simulink model "shuzi"  (Simulink 5.0)
settings: Solver=ode45  StartTime=0.0  StopTime=10.0  RelTol=1e-3
undefined symbols (not defined in the file): rcosine
libraries: dspsigops x6, simulink x3, commsink2 x2, commchan2 x1, commrandsrc2 x1, commutil2 x1, dspswit3 x1, dsparch4 x1, commcontsrc2 x1
settings Model: LastModifiedBy=lenovo

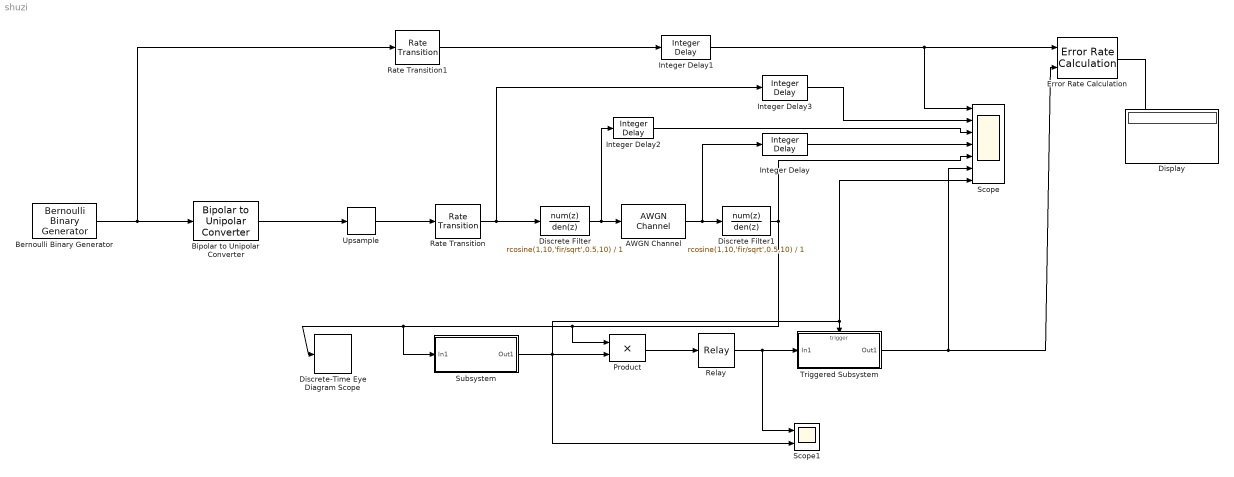
== system shuzi ==
  AWGN Channel : commchan2/AWGN Channel  seed=67  noiseMode=Variance from mask  EsNodB=10  SNRdB=10  Ps=1  Tsym=1  variance=0.05
  Bernoulli Binary Generator : commrandsrc2/Bernoulli Binary Generator  P=0.5  seed=67  Ts=0.001  frameBased=off  sampPerFrame=1  orient=off
  Bipolar to Unipolar Converter : commutil2/Bipolar to Unipolar Converter  M=2  polarity=Positive
  Discrete Filter : DiscreteFilter  Numerator=rcosine(1,10,'fir/sqrt',0.5,10)  Denominator=1  SampleTime=1/1e4
  Discrete Filter1 : DiscreteFilter  Numerator=rcosine(1,10,'fir/sqrt',0.5,10)  Denominator=1  SampleTime=1/1e4
  Discrete-Time Eye Diagram Scope : commsink2/Discrete-Time Eye Diagram Scope  Tag=EyeDiagram  showPlotting=on  sampPerSymb=10  offsetEye=0  symbPerTrace=1  numTraces=40  numNewFrames=10  showRendering=off  LineStyles=-  LineColors=b  dupPoints=on  fading=on  render=on  AxisGrid=on  showAxes=off  yMin=-0.307675209718084  yMax=6.47656316456567  inphaseLabel=In-phase Amplitude  quadratureLabel=Quadrature Amplitude  showFigure=off  openScopeAtSimStart=on  dispDiagram=In-phase and Quadrature  FrameNumber=off  FigPos=[520 166 560 644]  figTitle=Eye Diagram  block_type_=eye  numLinesMax=8
  Display : Display
  Error Rate Calculation : commsink2/Error Rate Calculation  N=0  st_delay=0  cp_mode=Entire frame  subframe=[]  PMode=Port  WsName=ErrorVec  RsMode2=off  stop=off  numErr=100  maxBits=1e6
  Integer Delay : dspsigops/Integer Delay  delay=100  ic=0  reset_popup=None
  Integer Delay1 : dspsigops/Integer Delay  delay=207  ic=0  reset_popup=None
  Integer Delay2 : dspsigops/Integer Delay  delay=100  ic=0  reset_popup=None
  Integer Delay3 : dspsigops/Integer Delay  delay=202  ic=0  reset_popup=None
  Product : Product  SaturateOnIntegerOverflow=on
  Rate Transition : simulink/Signal Attributes/Rate Transition  DataIntegrity=on  DeterministicTransfer=on  TransitionType=Slow to fast  InitCond=0
  Rate Transition1 : simulink/Signal Attributes/Rate Transition  DataIntegrity=on  DeterministicTransfer=on  TransitionType=Slow to fast  InitCond=0
  Relay : Relay  OnSwitchValue=0  OffSwitchValue=0
  Scope : Scope  NumInputPorts=7
      settings: TickLabels=on  YMin=0~0~0.6~-0.5~1~-2~0  YMax=1~1~1.8~2.5~7~2~1
  Scope1 : Scope  NumInputPorts=2
      settings: YMin=-5~-5  YMax=5~5
  Subsystem : Subsystem
  Triggered Subsystem : Subsystem  TreatAsAtomicUnit=on
  Upsample : dspsigops/Upsample  N=2  phase=0  ic=0  mode=Maintain input frame size
  wires:
  Bernoulli Binary Generator/1 -> Bipolar to Unipolar Converter/1, Rate Transition1/1
  Upsample/1 -> Rate Transition/1
  Rate Transition/1 -> Discrete Filter/1, Integer Delay3/1
  Rate Transition1/1 -> Integer Delay1/1
  Relay/1 -> Triggered Subsystem/1(In1), Scope1/1
  Product/1 -> Relay/1
  Subsystem/1(Out1) -> Product/2, Scope1/2, Triggered Subsystem/Trigger, Scope/7
  Integer Delay3/1 -> Scope/2
  Integer Delay2/1 -> Scope/3
  Integer Delay/1 -> Scope/4
  Error Rate Calculation/1 -> Display/1
  Integer Delay1/1 -> Error Rate Calculation/1, Scope/1
  Discrete Filter1/1 -> Discrete-Time Eye Diagram Scope/1, Subsystem/1(In1), Product/1, Scope/5
  Triggered Subsystem/1(Out1) -> Error Rate Calculation/2, Scope/6
  Bipolar to Unipolar Converter/1 -> Upsample/1
  AWGN Channel/1 -> Discrete Filter1/1, Integer Delay/1
  Discrete Filter/1 -> AWGN Channel/1, Integer Delay2/1

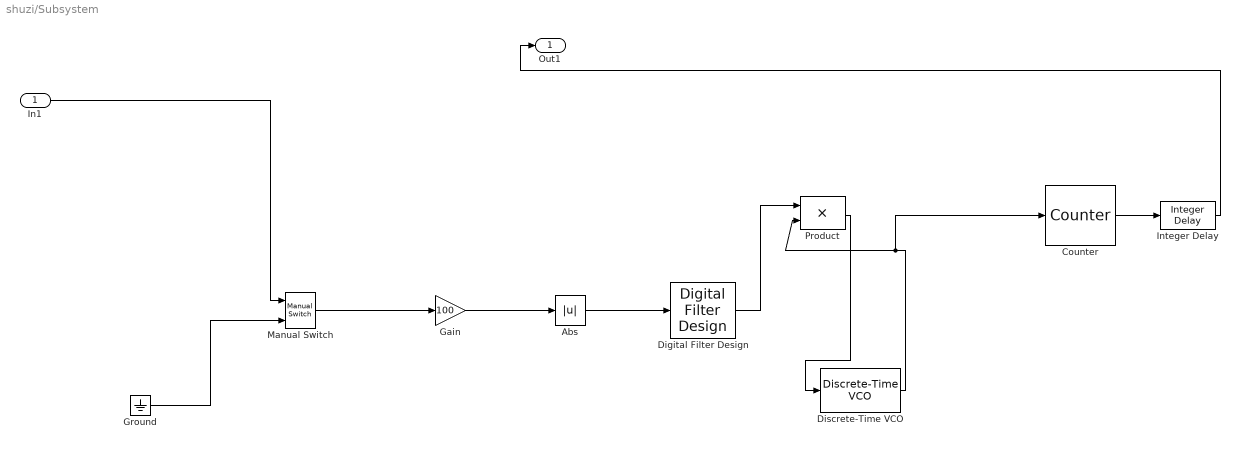
== system shuzi/Subsystem ==
  In1 : Inport
  Abs : Abs  SaturateOnIntegerOverflow=on
  Counter : dspswit3/Counter  Direction=Up  CountEvent=Non-zero sample  CounterSize=User defined  MaxCount=1  InitialCount=0  Output=Count  HitValue=32  ResetInput=off  SamplesPerFrame=1  Ts=1  CntDtype=Double  HitDtype=Logical
  Digital Filter Design : dsparch4/Digital Filter Design
  Discrete-Time VCO : commcontsrc2/Discrete-Time VCO  Ac=1  Fc=1994  Kc=8  Ph=0  ts=0.0001
  Gain : Gain  Gain=100  SaturateOnIntegerOverflow=on
  Ground : Ground
  Integer Delay : dspsigops/Integer Delay  delay=4  ic=0  reset_popup=None
  Manual Switch : simulink/Signal Routing/Manual Switch  sw=1  action=0
  Product : Product  SaturateOnIntegerOverflow=on
  Out1 : Outport
  wires:
  In1/1 -> Manual Switch/1
  Ground/1 -> Manual Switch/2
  Manual Switch/1 -> Gain/1
  Gain/1 -> Abs/1
  Abs/1 -> Digital Filter Design/1
  Digital Filter Design/1 -> Product/1
  Product/1 -> Discrete-Time VCO/1
  Discrete-Time VCO/1 -> Product/2, Counter/1
  Counter/1 -> Integer Delay/1
  Integer Delay/1 -> Out1/1

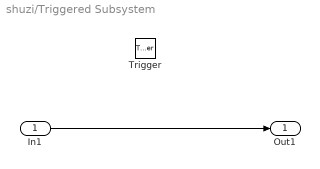
== system shuzi/Triggered Subsystem ==
  In1 : Inport
  Trigger : TriggerPort
  Out1 : Outport
  wires:
  In1/1 -> Out1/1
